simulink library "lib_rigid_body_kinematics"  (Simulink 8.5)
settings: Solver=ode45  StartTime=0.0  StopTime=10.0  RelTol=1e-3
undefined symbols (not defined in the file or in its folder): omega0_t0, quat_t0, r0, rD0, rotvec_t0, Ts
undefined symbols (not defined in the file): r_B_B_C, R_t0
libraries: lib_transformations x6, lib_rigid_body_kinematics x4
settings Model: Creator=schappler  LastModifiedBy=schappler

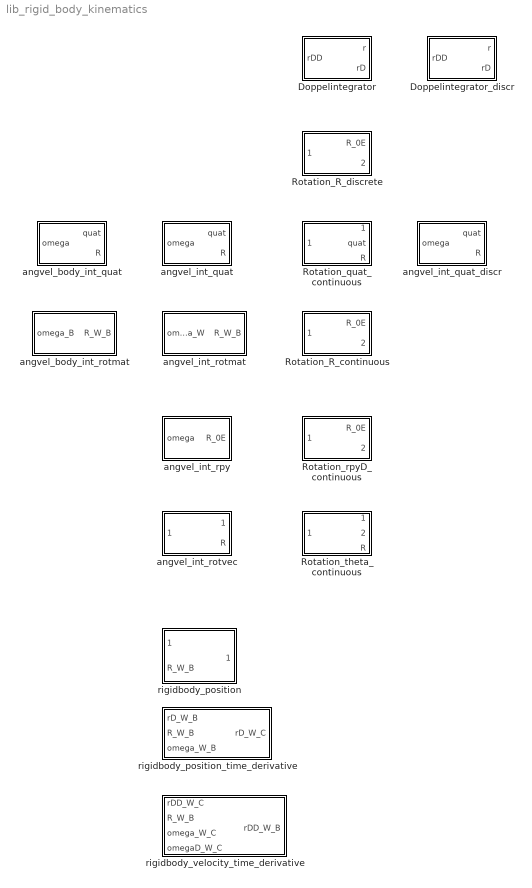
== system lib_rigid_body_kinematics ==
  Doppelintegrator : Subsystem  mask{r0=r0, rD0=rD0, Name_v='x'}
      mask prompts: r0 "Anfangsposition (3x1)"; rD0 "Anfangsgeschwindigkeit (3x1)"; Name_v "Name der Variablen (nur für Beschriftung)"
      mask Display:
      | port_label('input', 1, sprintf('%sDD', Name_v))
      | port_label('output', 1, sprintf('%s', Name_v))
      | port_label('output', 2, sprintf('%sD', Name_v))
  Doppelintegrator_discr : Subsystem  mask{r0=r0, rD0=rD0, Ts=Ts}
      mask prompts: r0 "Anfangsposition (3x1)"; rD0 "Anfangsgeschwindigkeit (3x1)"; Ts "Abtastzeit"
  Rotation_R_continuous : Subsystem  mask{R_0E_t0=R_t0, omega0_t0=omega0_t0}
      mask prompts: R_0E_t0 "Anfangsrotation (3x3)"; omega0_t0 "Anfangsdrehgeschwindigkeit (3x1)"
  Rotation_R_discrete : Subsystem  mask{R_0E_t0=R_t0, omega0_t0=omega0_t0, T=1e-3}
      mask prompts: R_0E_t0 "Anfangsrotation (3x3)"; omega0_t0 "Anfangsdrehgeschwindigkeit (3x1)"; T "Abtastzeit"
  Rotation_quat_continuous : Subsystem  mask{quat_t0=quat_t0, omega0_t0=omega0_t0}
      mask prompts: quat_t0 "Anfangsrotation (4x1) (Quaternion)"; omega0_t0 "Anfangsdrehgeschwindigkeit (3x1)"
  Rotation_rpyD_continuous : Subsystem  mask{R_0E_t0=R_t0, omega0_t0=omega0_t0}
      mask prompts: R_0E_t0 "Anfangsrotation (3x3)"; omega0_t0 "Anfangsdrehgeschwindigkeit (3x1)"
      mask init:
      | % Anfangswert für RPY-Winkel
      | rpy_t0 = r2rpy(R_0E_t0);
  Rotation_theta_continuous : Subsystem  mask{rotvec_t0=rotvec_t0, omega0_t0=omega0_t0}
      mask prompts: rotvec_t0 "Anfangsrotation (3x1) (Rotationsvektor)"; omega0_t0 "Anfangsdrehgeschwindigkeit (3x1)"
  angvel_body_int_quat : Subsystem  mask{quat_t0=quat_t0, KSName_B='B', KSName_W='W'}
      mask prompts: quat_t0 "Anfangsrotation (4x1) (Quaternion)"
      mask Display:
      | port_label('input', 1, sprintf('_{(%s)}\\omega_{%s,%s}', KSName_B, KSName_W, KSName_B), 'texmode', 'on')
      | port_label('output', 1, sprintf('quat'))
      | port_label('output', 2, sprintf('^{%s}R_%s', KSName_W, KSName_B), 'texmode', 'on')
  angvel_body_int_rotmat : Subsystem  mask{R_0E_t0=R_t0, KSName_W='W', KSName_B='B'}
      mask prompts: R_0E_t0 "Anfangsrotation (3x3)"
      mask Display:
      | port_label('input', 1, sprintf('_{(%s)}\\omega_{%s,%s}', KSName_B, KSName_W, KSName_B), 'texmode', 'on')
      | port_label('output', 1, sprintf('^{%s}R_%s', KSName_W, KSName_B), 'texmode', 'on')
  angvel_int_quat : Subsystem  mask{quat_t0=quat_t0, KSName_B='B', KSName_W='W'}
      mask prompts: quat_t0 "Anfangsrotation (4x1) (Quaternion)"
      mask Display:
      | port_label('input', 1, sprintf('_{(%s)}\\omega_{%s,%s}', KSName_W, KSName_W, KSName_B), 'texmode', 'on')
      | port_label('output', 1, sprintf('quat'))
      | port_label('output', 2, sprintf('^{%s}R_%s', KSName_W, KSName_B), 'texmode', 'on')
  angvel_int_quat_discr : Subsystem  mask{quat_t0=quat_t0, Ts=Ts}
      mask prompts: quat_t0 "Anfangsrotation (4x1) (Quaternion)"; Ts "Abtastzeit"
  angvel_int_rotmat : Subsystem  mask{R_0E_t0=R_t0, KSName_W='W', KSName_B='B'}
      mask prompts: R_0E_t0 "Anfangsrotation (3x3)"
      mask Display:
      | port_label('input', 1, sprintf('_{(%s)}\\omega_{%s,%s}', KSName_W, KSName_W, KSName_B), 'texmode', 'on')
      | port_label('output', 1, sprintf('^{%s}R_%s', KSName_W, KSName_B), 'texmode', 'on')
  angvel_int_rotvec : Subsystem  mask{rotvec_t0=rotvec_t0}
      mask prompts: rotvec_t0 "Anfangsrotation (3x1) (Rotationsvektor)"
  angvel_int_rpy : Subsystem  mask{R_0E_t0=R_t0}
      mask prompts: R_0E_t0 "Anfangsrotation (3x3)"
      mask init:
      | % Anfangswert für RPY-Winkel
      | rpy_t0 = r2rpy(R_0E_t0);
  rigidbody_position : Subsystem  mask{r_B_B_C=r_B_B_C, PktName_B='B', PktName_C='C', KSName_W='W'}
      mask prompts: r_B_B_C "Konstanter Vektor von Punkt B zu C"; PktName_B "Punktname B"; PktName_C "Punktname C"; KSName_W "Koordinatensystemname W"
      mask Display:
      | port_label('input', 1, sprintf('r_%s_%s', KSName_W, PktName_B))
      | port_label('input', 2, sprintf('R_%s_%s', KSName_W, PktName_B))
      | port_label('output', 1, sprintf('r_%s_%s', KSName_W, PktName_C))
  rigidbody_position_time_derivative : Subsystem  mask{r_B_B_C=r_B_B_C, PktName_B='B', PktName_C='C', KSName_W='W'}
      mask prompts: r_B_B_C "Konstanter Vektor von Punkt B zu C"; PktName_B "Punktname B"; PktName_C "Punktname C"; KSName_W "Koordinatensystemname W"
      mask Display:
      | port_label('input', 1, sprintf('rD_%s_%s', KSName_W, PktName_B))
      | port_label('input', 2, sprintf('R_%s_%s', KSName_W, PktName_B))
      | port_label('input', 3, sprintf('\\omega_{%s,%s}', KSName_W, PktName_B), 'texmode', 'on')
      | port_label('output', 1, sprintf('rD_%s_%s', KSName_W, PktName_C))
  rigidbody_velocity_time_derivative : Subsystem  mask{r_B_B_C=r_B_B_C, PktName_B='B', PktName_C='C', KSName_W='W'}
      mask prompts: r_B_B_C "Konstanter Vektor von Punkt B zu C"; PktName_B "Punktname B"; PktName_C "Punktname C"; KSName_W "Koordinatensystemname W"
      mask Display:
      | port_label('input', 1, sprintf('rDD_%s_%s', KSName_W, PktName_B))
      | port_label('input', 2, sprintf('R_%s_%s', KSName_W, PktName_B))
      | port_label('input', 3, sprintf('\\omega_{%s,%s}', KSName_W, PktName_B), 'texmode', 'on')
      | port_label('input', 4, sprintf('\\omegaD_{%s,%s}', KSName_W, PktName_B), 'texmode', 'on')
      | port_label('output', 1, sprintf('rDD_%s_%s', KSName_W, PktName_C))

== system lib_rigid_body_kinematics/Doppelintegrator ==
  note: Siehe: http://blogs.mathworks.com/simulink/2014/01/22/how-to-model-a-hard-stop-in-simulink/
      |
      | Dieser Block hat eigentlich keinen Mehrwert (bis auf die Maskierung des Variablennamens)
  rDD : Inport
  "Integrator, Second-Order" : SecondOrderIntegrator  ICX=r0  ICDXDT=rD0
  r : Outport
  rD : Outport  Port=2
  wires:
  rDD/1 -> "Integrator, Second-Order"/1
  "Integrator, Second-Order"/1 -> r/1
  "Integrator, Second-Order"/2 -> rD/1

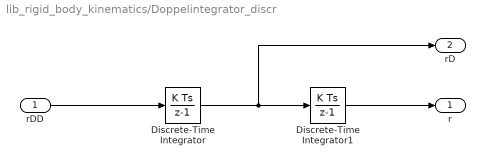
== system lib_rigid_body_kinematics/Doppelintegrator_discr ==
  rDD : Inport
  Discrete-Time Integrator : DiscreteIntegrator  InitialCondition=rD0  InitialConditionSetting=State (most efficient)  SampleTime=Ts
  Discrete-Time Integrator1 : DiscreteIntegrator  InitialCondition=r0  InitialConditionSetting=State (most efficient)  SampleTime=Ts
  r : Outport
  rD : Outport  Port=2
  wires:
  Discrete-Time Integrator/1 -> Discrete-Time Integrator1/1, rD/1
  rDD/1 -> Discrete-Time Integrator/1
  Discrete-Time Integrator1/1 -> r/1

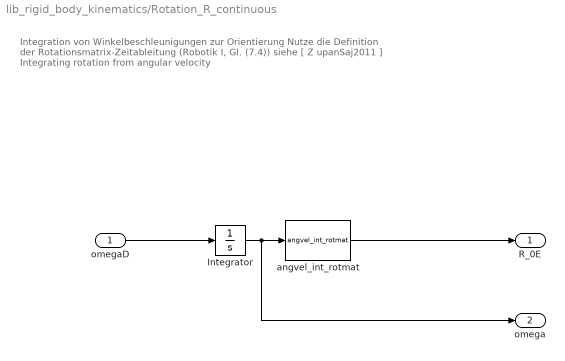
== system lib_rigid_body_kinematics/Rotation_R_continuous ==
  note: Integration von Winkelbeschleunigungen zur Orientierung
      | Nutze die Definition der Rotationsmatrix-Zeitableitung (Robotik I, Gl. (7.4))
      | siehe [ Z upanSaj2011 ] Integrating rotation from angular velocity
  omegaD : Inport  PortDimensions=3
  Integrator : Integrator  InitialCondition=omega0_t0
  angvel_int_rotmat : lib_rigid_body_kinematics/angvel_int_rotmat  R_0E_t0=R_t0  KSName_W='W'  KSName_B='B'
  R_0E : Outport  PortDimensions=[3 3]  SampleTime=0
  omega : Outport  Port=2  PortDimensions=3
  wires:
  Integrator/1 -> omega/1, angvel_int_rotmat/1
  omegaD/1 -> Integrator/1
  angvel_int_rotmat/1 -> R_0E/1

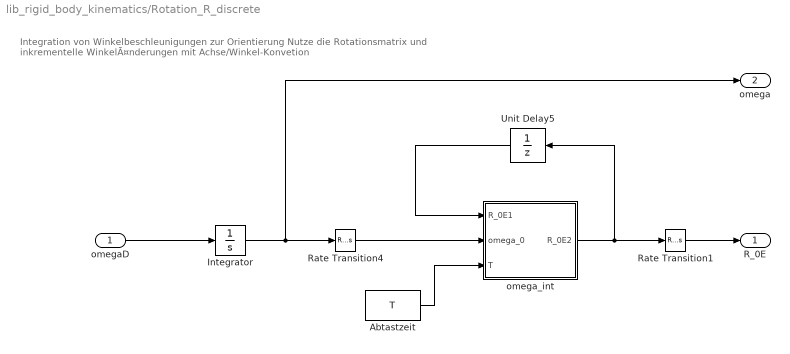
== system lib_rigid_body_kinematics/Rotation_R_discrete ==
  note: Integration von Winkelbeschleunigungen zur Orientierung
      | Nutze die Rotationsmatrix und inkrementelle WinkelÃ¤nderungen mit Achse/Winkel-Konvetion
  omegaD : Inport  PortDimensions=3
  Abtastzeit : Constant  Value=T
  Integrator : Integrator  InitialCondition=omega0_t0
  Rate Transition1 : RateTransition  OutPortSampleTime=0
  Rate Transition4 : RateTransition  OutPortSampleTime=T
  Unit Delay5 : UnitDelay  InitialCondition=R_0E_t0  SampleTime=-1
  omega_int : MATLAB Function  TreatAsAtomicUnit=on
  R_0E : Outport  PortDimensions=[3 3]  SampleTime=0
  omega : Outport  Port=2  PortDimensions=3
  wires:
  omegaD/1 -> Integrator/1
  Abtastzeit/1 -> omega_int/3(T)
  Integrator/1 -> omega/1, Rate Transition4/1
  omega_int/1(R_0E2) -> Unit Delay5/1, Rate Transition1/1
  Rate Transition4/1 -> omega_int/2(omega_0)
  Unit Delay5/1 -> omega_int/1(R_0E1)
  Rate Transition1/1 -> R_0E/1

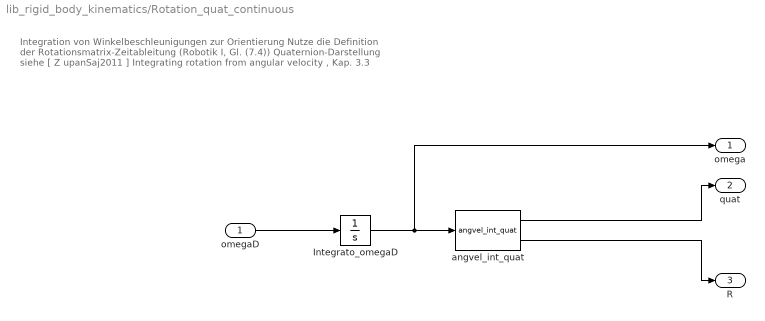
== system lib_rigid_body_kinematics/Rotation_quat_continuous ==
  note: Integration von Winkelbeschleunigungen zur Orientierung
      | Nutze die Definition der Rotationsmatrix-Zeitableitung (Robotik I, Gl. (7.4))
      | Quaternion-Darstellung
      | siehe [ Z upanSaj2011 ] Integrating rotation from angular velocity , Kap. 3.3
  omegaD : Inport  PortDimensions=3
  Integrato_omegaD : Integrator  InitialCondition=omega0_t0
  angvel_int_quat : lib_rigid_body_kinematics/angvel_int_quat  quat_t0=quat_t0
  omega : Outport  PortDimensions=3
  quat : Outport  Port=2  PortDimensions=4
  R : Outport  Port=3  PortDimensions=[3 3]
  wires:
  Integrato_omegaD/1 -> omega/1, angvel_int_quat/1
  omegaD/1 -> Integrato_omegaD/1
  angvel_int_quat/2 -> R/1
  angvel_int_quat/1 -> quat/1

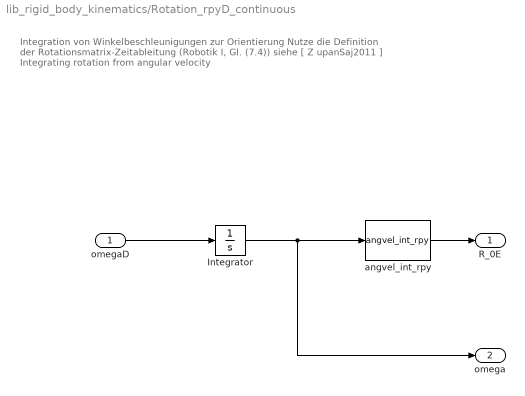
== system lib_rigid_body_kinematics/Rotation_rpyD_continuous ==
  note: Integration von Winkelbeschleunigungen zur Orientierung
      | Nutze die Definition der Rotationsmatrix-Zeitableitung (Robotik I, Gl. (7.4))
      | siehe [ Z upanSaj2011 ] Integrating rotation from angular velocity
  omegaD : Inport  PortDimensions=3
  Integrator : Integrator  InitialCondition=omega0_t0
  angvel_int_rpy : lib_rigid_body_kinematics/angvel_int_rpy  R_0E_t0=R_t0
  R_0E : Outport  PortDimensions=[3 3]  SampleTime=0
  omega : Outport  Port=2  PortDimensions=3
  wires:
  Integrator/1 -> omega/1, angvel_int_rpy/1
  omegaD/1 -> Integrator/1
  angvel_int_rpy/1 -> R_0E/1

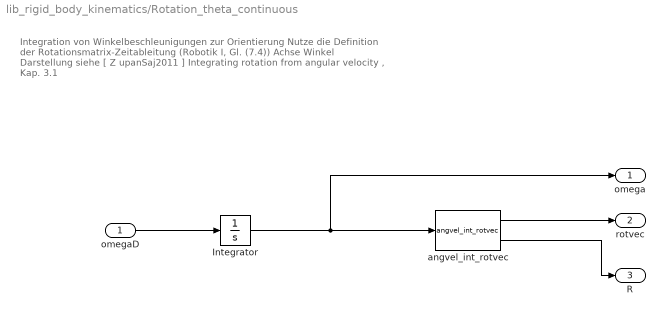
== system lib_rigid_body_kinematics/Rotation_theta_continuous ==
  note: Integration von Winkelbeschleunigungen zur Orientierung
      | Nutze die Definition der Rotationsmatrix-Zeitableitung (Robotik I, Gl. (7.4))
      | Achse Winkel Darstellung
      | siehe [ Z upanSaj2011 ] Integrating rotation from angular velocity , Kap. 3.1
  omegaD : Inport  PortDimensions=3
  Integrator : Integrator  InitialCondition=omega0_t0
  angvel_int_rotvec : lib_rigid_body_kinematics/angvel_int_rotvec  rotvec_t0=rotvec_t0
  omega : Outport  PortDimensions=3
  rotvec : Outport  Port=2  PortDimensions=3
  R : Outport  Port=3  PortDimensions=[3 3]
  wires:
  Integrator/1 -> omega/1, angvel_int_rotvec/1
  omegaD/1 -> Integrator/1
  angvel_int_rotvec/2 -> R/1
  angvel_int_rotvec/1 -> rotvec/1

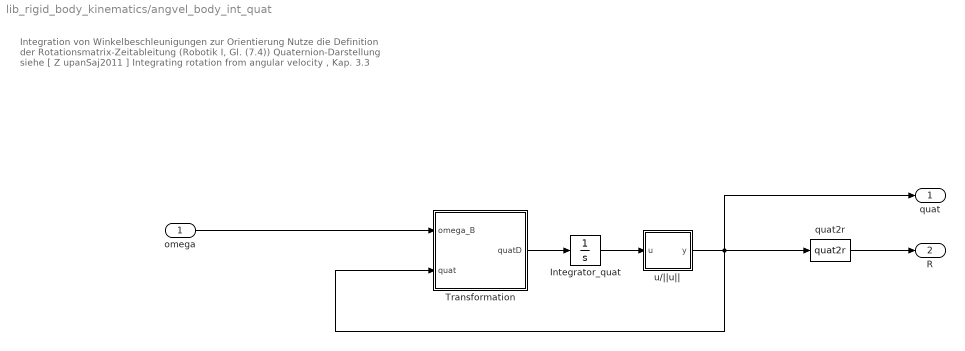
== system lib_rigid_body_kinematics/angvel_body_int_quat ==
  note: Integration von Winkelbeschleunigungen zur Orientierung
      | Nutze die Definition der Rotationsmatrix-Zeitableitung (Robotik I, Gl. (7.4))
      | Quaternion-Darstellung
      | siehe [ Z upanSaj2011 ] Integrating rotation from angular velocity , Kap. 3.3
  omega : Inport  PortDimensions=3
  Integrator_quat : Integrator  InitialCondition=quat_t0
  Transformation : MATLAB Function  TreatAsAtomicUnit=on
  quat2r : lib_transformations/quat2r
  u/||u|| : MATLAB Function  TreatAsAtomicUnit=on
  quat : Outport  PortDimensions=4
  R : Outport  Port=2  PortDimensions=[3 3]
  wires:
  Integrator_quat/1 -> u/||u||/1(u)
  omega/1 -> Transformation/1(omega_B)
  Transformation/1(quatD) -> Integrator_quat/1
  quat2r/1 -> R/1
  u/||u||/1(y) -> quat/1, quat2r/1, Transformation/2(quat)

== system lib_rigid_body_kinematics/angvel_body_int_rotmat ==
  note: Integration von Winkelbeschleunigungen zur Orientierung
      | Nutze die Definition der Rotationsmatrix-Zeitableitung (Robotik I, Gl. (7.4))
      | siehe [ Z upanSaj2011 ] Integrating rotation from angular velocity; Equ. (5)
      |
      | Eingabe: Winkelgeschwindigkeit im Körper-KS (mitgedreht)
  omega_B : Inport  PortDimensions=3
  Integrator1 : Integrator  InitialCondition=R_0E_t0
  Product : Product  Multiplication=Matrix(*)
  skew : lib_transformations/skew
  R_W_B : Outport  PortDimensions=[3 3]  SampleTime=0
  wires:
  Integrator1/1 -> Product/1, R_W_B/1
  skew/1 -> Product/2
  omega_B/1 -> skew/1
  Product/1 -> Integrator1/1

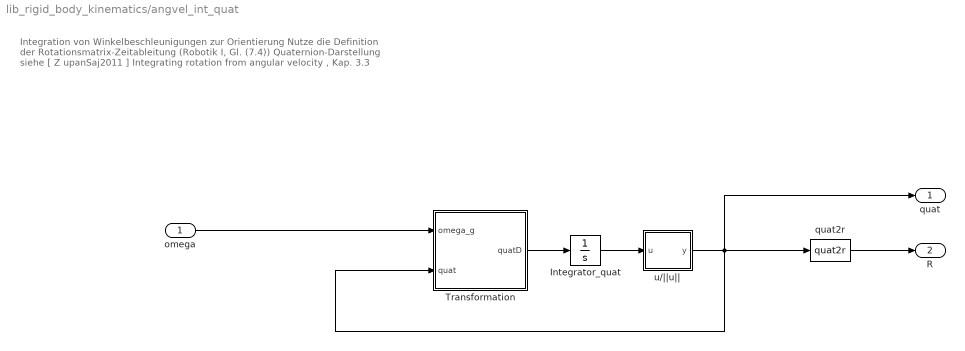
== system lib_rigid_body_kinematics/angvel_int_quat ==
  note: Integration von Winkelbeschleunigungen zur Orientierung
      | Nutze die Definition der Rotationsmatrix-Zeitableitung (Robotik I, Gl. (7.4))
      | Quaternion-Darstellung
      | siehe [ Z upanSaj2011 ] Integrating rotation from angular velocity , Kap. 3.3
  omega : Inport  PortDimensions=3
  Integrator_quat : Integrator  InitialCondition=quat_t0
  Transformation : MATLAB Function  TreatAsAtomicUnit=on
  quat2r : lib_transformations/quat2r
  u/||u|| : MATLAB Function  TreatAsAtomicUnit=on
  quat : Outport  PortDimensions=4
  R : Outport  Port=2  PortDimensions=[3 3]
  wires:
  Integrator_quat/1 -> u/||u||/1(u)
  omega/1 -> Transformation/1(omega_g)
  Transformation/1(quatD) -> Integrator_quat/1
  quat2r/1 -> R/1
  u/||u||/1(y) -> quat/1, quat2r/1, Transformation/2(quat)

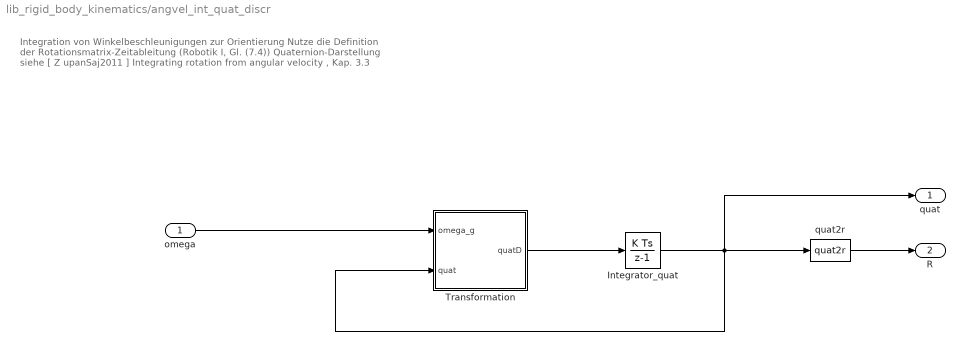
== system lib_rigid_body_kinematics/angvel_int_quat_discr ==
  note: Integration von Winkelbeschleunigungen zur Orientierung
      | Nutze die Definition der Rotationsmatrix-Zeitableitung (Robotik I, Gl. (7.4))
      | Quaternion-Darstellung
      | siehe [ Z upanSaj2011 ] Integrating rotation from angular velocity , Kap. 3.3
  omega : Inport  PortDimensions=3
  Integrator_quat : DiscreteIntegrator  InitialCondition=quat_t0  InitialConditionSetting=State (most efficient)  SampleTime=Ts
  Transformation : MATLAB Function  TreatAsAtomicUnit=on
  quat2r : lib_transformations/quat2r
  quat : Outport  PortDimensions=4
  R : Outport  Port=2  PortDimensions=[3 3]
  wires:
  Integrator_quat/1 -> quat2r/1, quat/1, Transformation/2(quat)
  omega/1 -> Transformation/1(omega_g)
  Transformation/1(quatD) -> Integrator_quat/1
  quat2r/1 -> R/1

== system lib_rigid_body_kinematics/angvel_int_rotmat ==
  note: Integration von Winkelbeschleunigungen zur Orientierung
      | Nutze die Definition der Rotationsmatrix-Zeitableitung (Robotik I, Gl. (7.4))
      | siehe [ Z upanSaj2011 ] Integrating rotation from angular velocity; Equ. (4)
      |
      | Eingabe: Winkelgeschwindigkeit im Welt-KS (fix)
  omega_W : Inport  PortDimensions=3
  Integrator1 : Integrator  InitialCondition=R_0E_t0
  Product : Product  Multiplication=Matrix(*)
  skew : lib_transformations/skew
  R_W_B : Outport  PortDimensions=[3 3]  SampleTime=0
  wires:
  Integrator1/1 -> Product/2, R_W_B/1
  skew/1 -> Product/1
  omega_W/1 -> skew/1
  Product/1 -> Integrator1/1

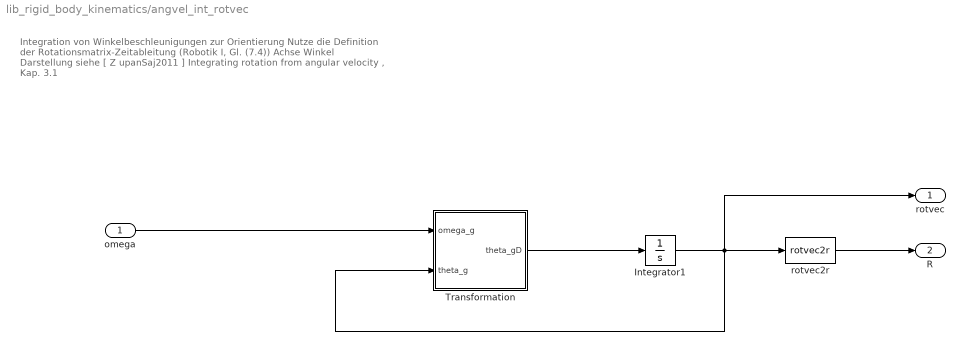
== system lib_rigid_body_kinematics/angvel_int_rotvec ==
  note: Integration von Winkelbeschleunigungen zur Orientierung
      | Nutze die Definition der Rotationsmatrix-Zeitableitung (Robotik I, Gl. (7.4))
      | Achse Winkel Darstellung
      | siehe [ Z upanSaj2011 ] Integrating rotation from angular velocity , Kap. 3.1
  omega : Inport  PortDimensions=3
  Integrator1 : Integrator  InitialCondition=rotvec_t0
  Transformation : MATLAB Function  TreatAsAtomicUnit=on
  rotvec2r : lib_transformations/rotvec2r
  rotvec : Outport  PortDimensions=3
  R : Outport  Port=2  PortDimensions=[3 3]
  wires:
  Integrator1/1 -> rotvec2r/1, rotvec/1, Transformation/2(theta_g)
  Transformation/1(theta_gD) -> Integrator1/1
  rotvec2r/1 -> R/1
  omega/1 -> Transformation/1(omega_g)

== system lib_rigid_body_kinematics/angvel_int_rpy ==
  note: Integration von Winkelbeschleunigungen zur Orientierung
      | Nutze die Definition der Rotationsmatrix-Zeitableitung (Robotik I, Gl. (7.4))
      | siehe [ Z upanSaj2011 ] Integrating rotation from angular velocity
  omega : Inport  PortDimensions=3
  Integrator1 : Integrator  InitialCondition=rpy_t0
  omega2rpyD : MATLAB Function  TreatAsAtomicUnit=on
  rpy2r : MATLAB Function  TreatAsAtomicUnit=on
  R_0E : Outport  PortDimensions=[3 3]  SampleTime=0
  wires:
  omega/1 -> omega2rpyD/1(omega_0)
  omega2rpyD/1(rpyD) -> Integrator1/1
  Integrator1/1 -> rpy2r/1(rpy), omega2rpyD/2(rpy)
  rpy2r/1(R) -> R_0E/1

== system lib_rigid_body_kinematics/rigidbody_position ==
  r_W_W_B : Inport
  R_W_B : Inport  Port=2  PortDimensions=[3 3]
  MATLAB Function : MATLAB Function  TreatAsAtomicUnit=on
  r_W_W_C : Outport
  wires:
  R_W_B/1 -> MATLAB Function/2(R_W_B)
  r_W_W_B/1 -> MATLAB Function/1(r_W_W_B)
  MATLAB Function/1(r_W_W_C) -> r_W_W_C/1

== system lib_rigid_body_kinematics/rigidbody_position_time_derivative ==
  rD_W_B : Inport
  R_W_B : Inport  Port=2  PortDimensions=[3 3]
  omega_W_B : Inport  Port=3
  position_time_derivative_Fcn : MATLAB Function  TreatAsAtomicUnit=on
  rD_W_C : Outport
  wires:
  position_time_derivative_Fcn/1(rD_W_C) -> rD_W_C/1
  omega_W_B/1 -> position_time_derivative_Fcn/3(omega_W_B)
  rD_W_B/1 -> position_time_derivative_Fcn/1(rD_W_B)
  R_W_B/1 -> position_time_derivative_Fcn/2(R_W_B)

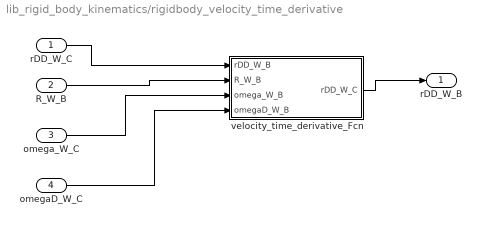
== system lib_rigid_body_kinematics/rigidbody_velocity_time_derivative ==
  rDD_W_C : Inport
  R_W_B : Inport  Port=2  PortDimensions=[3 3]
  omega_W_C : Inport  Port=3
  omegaD_W_C : Inport  Port=4
  velocity_time_derivative_Fcn : MATLAB Function  TreatAsAtomicUnit=on
  rDD_W_B : Outport
  wires:
  velocity_time_derivative_Fcn/1(rDD_W_C) -> rDD_W_B/1
  omega_W_C/1 -> velocity_time_derivative_Fcn/3(omega_W_B)
  rDD_W_C/1 -> velocity_time_derivative_Fcn/1(rDD_W_B)
  omegaD_W_C/1 -> velocity_time_derivative_Fcn/4(omegaD_W_B)
  R_W_B/1 -> velocity_time_derivative_Fcn/2(R_W_B)

== matlab function Rotation_R_discrete/omega_int ==
  data: R_0E1 input double; omega_0 input double; R_0E2 output double; T input double
% Integriere die Winkelgeschwindigkeit zu einer Winkelposition
% 
% Eingang:
% R_0E1
% omega_0
% T
%   Integrationsschrittweite
% Quellen:
% [1] Robotik I Skript

function R_0E2 = omega_int(R_0E1, omega_0, T)
%% Init
%#codegen
assert(isa(R_0E1,'double') && isreal(R_0E1) && all(size(R_0E1) == [3 3]), ...
  'Rotationsmatrix muss [3x3] double sein.');
assert(isa(omega_0,'double') && isreal(omega_0) && all(size(omega_0) == [3 1]), ...
  'Drehgeschwindigkeit muss [3x1] double sein.');
assert(isa(T,'double') && isreal(T) && all(size(T) == [1 1]), ...
  'Abtastzeit muss [1x1] double sein.');

%% Berechnung

% Drehgeschwindigkeit in KÃ¶rper-KS
omega_E = R_0E1' * omega_0;
% Drehwinkel
theta = norm(omega_E) * T;

if theta == 0
  % keine Drehung
  R_0E2 = R_0E1;
else
  % Drehachse
  v = omega_E / norm(omega_E);

  % Rotationsmatrix aus Achse-Winkel-Darstellung
  R_E_Ed = angvec2r(theta, v);
  
  % Neue Endpunkt-Rotationsmatrix
  R_0E2 = R_0E1 * R_E_Ed;
end

== matlab function angvel_int_quat_discr/Transformation ==
  data: omega_g input double; quat input double; quatD output double
% Integriere die Winkelgeschwindigkeit zu einer Winkelposition
% 
% Eingang:
% quat
%   Quaternion entsprechend der Rotationsmatrix R
% omega_G
%   Drehgeschwindigkeit im Bezugs-KS G
% 
% Ausgang:
% quatD
%   Zeitableitung Quaternion
% 
% Quellen:
% [ZupanSaj2011] Integrating rotation from angular velocity (2011)

% Moritz Schappler, schappler@irt.uni-hannover.de, 2016-02
% (c) Institut für Regelungstechnik, Universität Hannover

function quatD = transform(omega_g, quat)
%% Init
%#codegen
assert(isa(omega_g,'double') && isreal(omega_g) && all(size(omega_g) == [3 1]), ...
  'Drehgeschwindigkeit muss [3x1] double sein.');
assert(isa(quat,'double') && isreal(quat) && all(size(quat) == [4 1]), ...
  'Quaternion muss [4x1] double sein.');

%% Berechnung mit Quaternionen-Klasse
Quat = Quaternion(quat);
QuatD = dot(Quat, omega_g);
quatD = [QuatD.s; QuatD.v'];

%% Eigene Berechnung (nicht weiter vefolgt.)
% [ZupanSaj2011] S. 726
% omega_g_hat = [0; omega_g];
% Omega_g_hat = Quaternion(omega_g_hat);
% % [ZupanSaj2011] Gl. (19)
% quatD = 0.5 * Omega_g_hat * ...

== matlab function angvel_int_rpy/omega2rpyD ==
  data: omega_0 input double; rpyD output double; rpy input double
% Integriere die Winkelgeschwindigkeit zu einer Winkelposition
% 
% Eingang:
% omega_0
% Quellen:
% irt_matlabtoolbox/maple_codegen/rotation_rpy_omega.mw
% (generated file rpyD_from_omega.m)

function rpyD = omega2rpyD(omega_0, rpy)
%% Init
%#codegen
assert(isa(omega_0,'double') && isreal(omega_0) && all(size(omega_0) == [3 1]), ...
  'Drehgeschwindigkeit muss [3x1] double sein.');
assert(isa(rpy,'double') && isreal(rpy) && all(size(rpy) == [3 1]), ...
  'rpy-Winkel muessen [3x1] double sein.');

alpha_s=rpy(1);
beta_s=rpy(2);
wx=omega_0(1);
wy=omega_0(2);
wz=omega_0(3);

%% Berechnung
t115 = sin(alpha_s);
t116 = cos(alpha_s);
t119 = -wy * t115 + wz * t116;
t118 = cos(beta_s);
t114 = 0.1e1 / t118;
rpyD = [-(-t118 * wx + t119 * sin(beta_s)) * t114; wz * t115 + t116 * wy; t119 * t114;];

== matlab function rigidbody_position_time_derivative/position_time_derivative_Fcn ==
  data: rD_W_C output double; rD_W_B input double; R_W_B input double; omega_W_B input double; r_B_B_C parameter double
% Berechnung der Geschwindigkeit eines Punktes auf einem Starrkörper
% 
% Eingabe:
% rD_W_B
%   Geschwindigkeit des Punktes B (kann, muss nicht Basis des Körper-KS sein)
% R_W_B
%   Rotationsmatrix vom KS W (Welt) zum KS B (Körper)
% omega_W_B
%   Winkelgeschwindigkeit des Starrkörpers im Welt-Koordinatensystem W
% r_B_B_C
%   Konstanter Vektor vom körperfesten Punkt B zum körperfesten Punkt C
% 
% Ausgabe:
% rD_W_C
%   Geschwindigkeit des Punktes C (kann, muss nicht Schwerpunkt sein)
% 
% Quelle:
% [1] Ortmaier: Skript Robotik I
% 
% Moritz Schappler, schappler@irt.uni-hannover.de, 2016-03
% (c) Institut für Regelungstechnik, Universität Hannover

function rD_W_C = fcn(rD_W_B, R_W_B, omega_W_B, r_B_B_C)
%#codegen

r_W_B_C = R_W_B * r_B_B_C;
% [1], Gl. (7.17)
rD_W_C = rD_W_B + cross(omega_W_B, r_W_B_C);

== matlab function angvel_int_rotvec/Transformation ==
  data: omega_g input double; theta_g input double; theta_gD output double
% Integriere die Winkelgeschwindigkeit zu einer Winkelposition
% 
% Eingang:
% theta_g
%   Rotationsvektor (Achse-Winkel)
% omega_G
%   Drehgeschwindigkeit im Bezugs-KS G
% R
%   Rotationsmatrix von G (global) nach g (kÃ¶rperfest)
% 
% Ausgang:
% theta_gD
%   Zeitableitung Rotationsvektor (Achse-Winkel)
% 
% Quellen:
% [ZupanSaj2011] Integrating rotation from angular velocity (2011)

function theta_gD = transform(omega_g, theta_g)
%% Init
%#codegen
assert(isa(theta_g,'double') && isreal(theta_g) && all(size(theta_g) == [3 1]), ...
  'Rotationsvektor muss [3x1] double sein.');
assert(isa(omega_g,'double') && isreal(omega_g) && all(size(omega_g) == [3 1]), ...
  'Drehgeschwindigkeit muss [3x1] double sein.');

% [ZupanSaj2011] 

%% Berechnung
theta = norm(theta_g);
Theta_g = skew(theta_g);
% [ZupanSaj2011], equ. (8)
if theta == 0
  T_inv = eye(3);
else
  T_inv = eye(3) - 0.5* Theta_g + 1/theta^2*(1-theta/(2*tan(theta/2)))*Theta_g^2;
end
% [ZupanSaj2011], equ. (7)
theta_gD = T_inv * omega_g;

== matlab function rigidbody_velocity_time_derivative/velocity_time_derivative_Fcn ==
  data: rDD_W_B input double; R_W_B input double; rDD_W_C output double; omega_W_B input double; omegaD_W_B input double; r_B_B_C parameter double
% Berechnung der Beschleunigung eines Punktes auf einem Starrkörper
% 
% Eingabe:
% rDD_W_B
%   Beschleunigung des Punktes B (kann, muss nicht Basis des Körper-KS sein)
% R_W_B
%   Rotationsmatrix vom KS W (Welt) zum KS B (Körper)
% omega_W_B
%   Winkelgeschwindigkeit des Starrkörpers im Welt-Koordinatensystem W
% omegaD_W_B
%   Winkelbeschleunigung des Starrkörpers im Welt-Koordinatensystem W
% r_B_B_C
%   Konstanter Vektor vom körperfesten Punkt B zum körperfesten Punkt C
% 
% Ausgabe:
% rDD_W_C
%   Beschleunigung des Punktes C (kann, muss nicht Schwerpunkt sein)
% 
% Quelle:
% [1] Ortmaier: Skript Robotik I
% 
% Moritz Schappler, schappler@irt.uni-hannover.de, 2016-03
% (c) Institut für Regelungstechnik, Universität Hannover

function rDD_W_C = fcn(rDD_W_B, R_W_B, omega_W_B, omegaD_W_B , r_B_B_C)
%#codegen

r_W_B_C = R_W_B * r_B_B_C;
% [1], Gl. (7.18)
rDD_W_C = rDD_W_B + cross(omegaD_W_B, r_W_B_C) + ...
  cross(omega_W_B, cross(omega_W_B, r_W_B_C));

== matlab function angvel_int_quat/Transformation ==
  data: omega_g input double; quat input double; quatD output double
% Integriere die Winkelgeschwindigkeit zu einer Winkelposition
% 
% Eingang:
% quat
%   Quaternion entsprechend der Rotationsmatrix R
% omega_G
%   Drehgeschwindigkeit im Bezugs-KS G
% 
% Ausgang:
% quatD
%   Zeitableitung Quaternion
% 
% Quellen:
% [ZupanSaj2011] Integrating rotation from angular velocity (2011)

% Moritz Schappler, schappler@irt.uni-hannover.de, 2016-02
% (c) Institut für Regelungstechnik, Universität Hannover

function quatD = transform(omega_g, quat)
%% Init
%#codegen
assert(isa(omega_g,'double') && isreal(omega_g) && all(size(omega_g) == [3 1]), ...
  'Drehgeschwindigkeit muss [3x1] double sein.');
assert(isa(quat,'double') && isreal(quat) && all(size(quat) == [4 1]), ...
  'Quaternion muss [4x1] double sein.');

%% Berechnung mit Quaternionen-Klasse
Quat = Quaternion(quat);
QuatD = dot(Quat, omega_g);
quatD = [QuatD.s; QuatD.v'];

%% Eigene Berechnung (nicht weiter vefolgt.)
% [ZupanSaj2011] S. 726
% omega_g_hat = [0; omega_g];
% Omega_g_hat = Quaternion(omega_g_hat);
% % [ZupanSaj2011] Gl. (19)
% quatD = 0.5 * Omega_g_hat * ...

== matlab function angvel_body_int_quat/Transformation ==
  data: omega_B input double; quat input double; quatD output double
% Integriere die Winkelgeschwindigkeit zu einer Winkelposition
% 
% Eingang:
% quat
%   Quaternion entsprechend der Rotationsmatrix R
% omega_g
%   Drehgeschwindigkeit im mitgedrehten KS B
% 
% Ausgang:
% quatD
%   Zeitableitung Quaternion
% 
% Quellen:
% [ZupanSaj2011] Integrating rotation from angular velocity (2011)

% Moritz Schappler, schappler@irt.uni-hannover.de, 2017-07
% (c) Institut für Regelungstechnik, Universität Hannover

function quatD = transform(omega_B, quat)
%% Init
%#codegen
assert(isa(omega_B,'double') && isreal(omega_B) && all(size(omega_B) == [3 1]), ...
  'Drehgeschwindigkeit muss [3x1] double sein.');
assert(isa(quat,'double') && isreal(quat) && all(size(quat) == [4 1]), ...
  'Quaternion muss [4x1] double sein.');

%% Berechnung mit Quaternionen-Klasse
Quat = Quaternion(quat);
% TODO: Bessere "Quaternionen-Formel"
R_W_B = quat2r(quat');
QuatD = dot(Quat, R_W_B*omega_B);
quatD = [QuatD.s; QuatD.v'];

%% Eigene Berechnung (nicht weiter vefolgt.)
% [ZupanSaj2011] S. 726
% omega_g_hat = [0; omega_g];
% Omega_g_hat = Quaternion(omega_g_hat);
% % [ZupanSaj2011] Gl. (19)
% quatD = 0.5 * Omega_g_hat * ...

== matlab function angvel_int_rpy/rpy2r ==
  data: rpy input double; R output double
function R = rpy2r(rpy)
%% Init
%#codegen
assert(isa(rpy,'double') && isreal(rpy) && all(size(rpy) == [3 1]), ...
  'rpy-Winkel muessen [3x1] double sein.');

%% Berechnung
R=rpy2r(rpy(1), rpy(2), rpy(3));

== matlab function rigidbody_position/MATLAB Function ==
  data: r_W_W_B input double; r_W_W_C output double; R_W_B input double; r_B_B_C parameter double
function r_W_W_C = fcn(r_W_W_B, R_W_B, r_B_B_C)
%#codegen
r_W_B_C = R_W_B * r_B_B_C;
r_W_W_C = r_W_W_B + r_W_B_C;

== matlab function angvel_int_quat/u//||u|| ==
  data: u input double; y output double
function y = normalize(u)
%#codegen

y = u./norm(u);

== matlab function angvel_body_int_quat/u//||u|| ==
  data: u input double; y output double
function y = normalize(u)
%#codegen

y = u./norm(u);
